simulink model "Model2"  (R2021a)
settings: Solver=VariableStepAuto  StartTime=0.0  StopTime=10.0  RelTol=1e-3
settings Model: Creator=ameya  LastModifiedBy=ameya

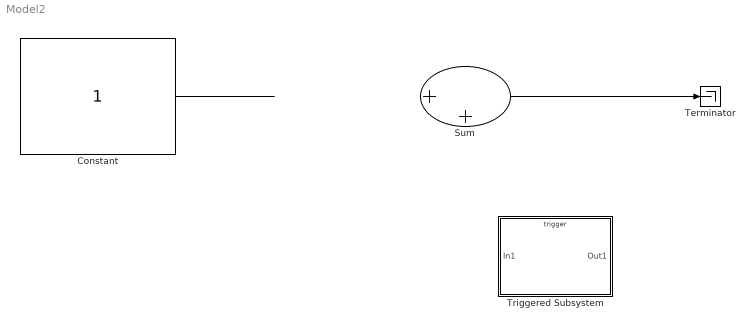
== system Model2 ==
  Constant : Constant
  Sum : Sum  Inputs=|++
  Terminator : Terminator
  Triggered Subsystem : Subsystem  TreatAsAtomicUnit=on
  wires:
  Constant/1 -> ?
  Sum/1 -> Terminator/1
  ? -> Triggered Subsystem/1(In1)

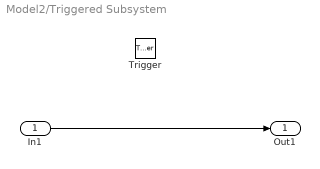
== system Model2/Triggered Subsystem ==
  In1 : Inport
  Trigger : TriggerPort  VariantControl=(inherit)
  Out1 : Outport
  wires:
  In1/1 -> Out1/1
